simulink model "NED_INS_V2"  (R2020a)
settings: Solver=FixedStepDiscrete  StartTime=0.0  StopTime=60  FixedStep=0.01  RelTol=1e-3
InitFcn:
  | INS_sample_time=0.01;
  | load('GPS1hz_INS_Car_60s.mat')
settings Model: Creator=Toranj  LastModifiedBy=Toranj

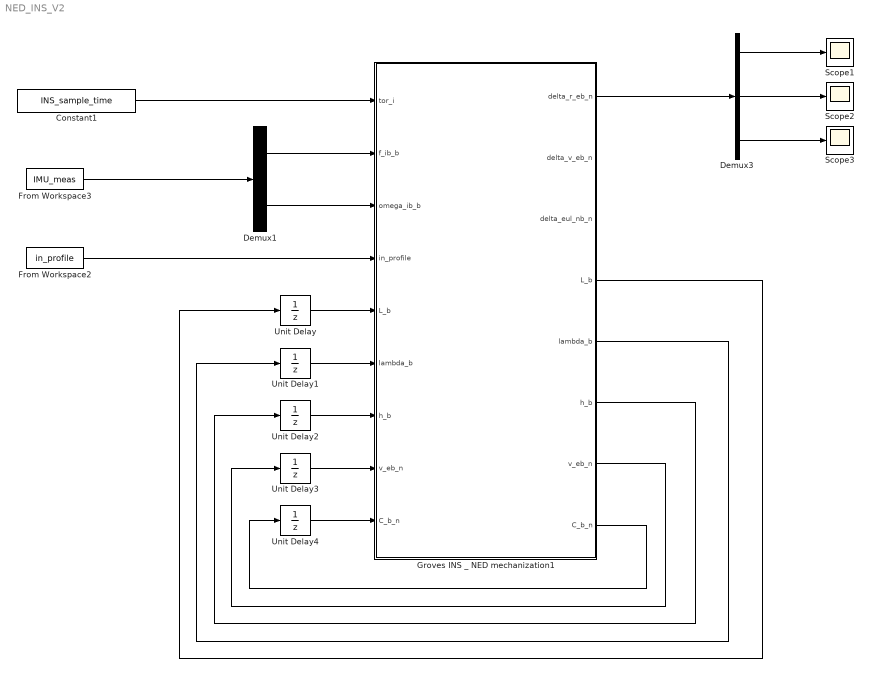
== system NED_INS_V2 ==
  Constant1 : Constant  Value=INS_sample_time
  Demux1 : Demux  Outputs=2
  Demux3 : Demux  Outputs=3
  From Workspace2 : FromWorkspace  VariableName=in_profile
  From Workspace3 : FromWorkspace  VariableName=IMU_meas
  Groves INS _ NED mechanization1 : MATLAB Function  TreatAsAtomicUnit=on  mask{old_true_L_b=0.890117918520000, old_true_lambda_b=0, old_true_h_b=10, old_true_v_eb_n=[0;0;0], old_true_C_b_n=eye(3)}
      mask prompts: old_true_L_b "Init_L_b"; old_true_lambda_b "Init_lambda_b"; old_true_h_b "Init_h_b"; old_true_v_eb_n "Init_v_eb_n"; old_true_C_b_n "Init_true_C_b_n"
      mask init:
      | deg_to_rad = 0.01745329252;
      | % rad_to_deg = 1/deg_to_rad;
      | % micro_g_to_meters_per_second_squared = 9.80665E-6;
      | 
      | % Position initialization error (m; N,E,D)
      | initialization_errors.delta_r_eb_n = [4;2;3];
      | % Velocity initialization error (m/s; N,E,D)
      | initialization_errors.delta_v_eb_n = [0.05;-0.05;0.1];
      | % Attitude initialization error (deg, converted to rad; @N,E,D)
      | initialization_errors.delta_eul_nb_n = [-0.05;0.04;1]*deg_to_rad; % rad
      | 
      | [L_b0,lambda_b0,h_b0,v_eb_n0,C_b_n0] =...
      |     Initialize_NED(old_true_L_b,old_true_lambda_b,old_true_h_b,...
      |     old_true_v_eb_n,old_true_C_b_n,initialization_errors);
  Scope1 : Scope
  Scope2 : Scope
  Scope3 : Scope
  Unit Delay : UnitDelay  InitialCondition=0.890117918520000  SampleTime=-1  HasFrameUpgradeWarning=on
  Unit Delay1 : UnitDelay  SampleTime=-1  HasFrameUpgradeWarning=on
  Unit Delay2 : UnitDelay  InitialCondition=10  SampleTime=-1  HasFrameUpgradeWarning=on
  Unit Delay3 : UnitDelay  InitialCondition=[0;0;0]  SampleTime=-1  HasFrameUpgradeWarning=on
  Unit Delay4 : UnitDelay  InitialCondition=eye(3)  SampleTime=-1  HasFrameUpgradeWarning=on
  wires:
  From Workspace2/1 -> Groves INS _ NED mechanization1/4(in_profile)
  Constant1/1 -> Groves INS _ NED mechanization1/1(tor_i)
  Demux1/1 -> Groves INS _ NED mechanization1/2(f_ib_b)
  From Workspace3/1 -> Demux1/1
  Unit Delay/1 -> Groves INS _ NED mechanization1/5("L_b ")
  Groves INS _ NED mechanization1/5(lambda_b) -> Unit Delay1/1
  Unit Delay2/1 -> Groves INS _ NED mechanization1/7("h_b ")
  Groves INS _ NED mechanization1/4(L_b) -> Unit Delay/1
  Groves INS _ NED mechanization1/8(C_b_n) -> Unit Delay4/1
  Unit Delay3/1 -> Groves INS _ NED mechanization1/8("v_eb_n ")
  Groves INS _ NED mechanization1/6(h_b) -> Unit Delay2/1
  Unit Delay1/1 -> Groves INS _ NED mechanization1/6("lambda_b ")
  Groves INS _ NED mechanization1/7(v_eb_n) -> Unit Delay3/1
  Unit Delay4/1 -> Groves INS _ NED mechanization1/9("C_b_n ")
  Demux1/2 -> Groves INS _ NED mechanization1/3(omega_ib_b)
  Demux3/3 -> Scope3/1
  Demux3/2 -> Scope2/1
  Demux3/1 -> Scope1/1
  Groves INS _ NED mechanization1/1(delta_r_eb_n) -> Demux3/1

== matlab function NED_INS_V2/Groves INS _ NED mechanization1 ==
  data: delta_r_eb_n output; delta_v_eb_n output; delta_eul_nb_n output; tor_i input; L_b output; f_ib_b input; omega_ib_b input; in_profile input; lambda_b output; h_b output; v_eb_n output; C_b_n output; L_b input; lambda_b input; h_b input; v_eb_n input; C_b_n input
% function [L_b,lambda_b,h_b,v_eb_n,C_b_n] = Nav_equations_NED(tor_i,...
%         old_L_b,old_lambda_b,old_h_b,old_v_eb_n,old_C_b_n,f_ib_b,omega_ib_b)
function [delta_r_eb_n,delta_v_eb_n,delta_eul_nb_n,L_b,lambda_b,h_b,v_eb_n,C_b_n] = Nav_equations_NED(tor_i,...
    f_ib_b,omega_ib_b,in_profile,L_b,lambda_b,h_b,v_eb_n,C_b_n)
%Nav_equations_NED - Runs precision local-navigation-frame inertial
%navigation equations (Note: only the attitude update and specific force
%frame transformation phases are precise.)
%
% Software for use with "Principles of GNSS, Inertial, and Multisensor
% Integrated Navigation Systems," Second Edition.
%
% This function created 1/4/2012 by Paul Groves
%
% Inputs:
%   tor_i         time interval between epochs (s)
%   old_L_b       previous latitude (rad)
%   old_lambda_b  previous longitude (rad)
%   old_h_b       previous height (m)
%   old_C_b_n     previous body-to-NED coordinate transformation matrix
%   old_v_eb_n    previous velocity of body frame w.r.t. ECEF frame, resolved
%                 along north, east, and down (m/s)
%   f_ib_b        specific force of body frame w.r.t. ECEF frame, resolved
%                 along body-frame axes, averaged over time interval (m/s^2)
%   omega_ib_b    angular rate of body frame w.r.t. ECEF frame, resolved
%                 about body-frame axes, averaged over time interval (rad/s)
% Outputs:
%   L_b           latitude (rad)
%   lambda_b      longitude (rad)
%   h_b           height (m)
%   v_eb_n        velocity of body frame w.r.t. ECEF frame, resolved along
%                 north, east, and down (m/s)
%   C_b_n         body-to-NED coordinate transformation matrix

% Copyright 2012, Paul Groves
% License: BSD; see license.txt for details

% parameters
omega_ie = 7.292115E-5;  % Earth rotation rate (rad/s)

% Begins
% persistent old_L_b old_lambda_b old_h_b old_v_eb_n old_C_b_n;
% if isempty(old_L_b)
%     old_L_b = L_b0;
%     old_lambda_b = lambda_b0;
%     old_h_b = h_b0;
%     old_v_eb_n = v_eb_n0;
%     old_C_b_n = C_b_n0;
% end
% PRELIMINARIES
% Calculate attitude increment, magnitude, and skew-symmetric matrix

    old_L_b = L_b;
    old_lambda_b = lambda_b;
    old_h_b = h_b;
    old_v_eb_n = v_eb_n;
    old_C_b_n = C_b_n;

alpha_ib_b = omega_ib_b * tor_i;
mag_alpha = sqrt(alpha_ib_b' * alpha_ib_b);
Alpha_ib_b = Skew_symmetric(alpha_ib_b);

% From (2.123) , determine the angular rate of the ECEF frame
% w.r.t the ECI frame, resolved about NED
omega_ie_n = omega_ie * [cos(old_L_b); 0; - sin(old_L_b)];

% From (5.44), determine the angular rate of the NED frame
% w.r.t the ECEF frame, resolved about NED
[old_R_N,old_R_E] = Radii_of_curvature(old_L_b);
old_omega_en_n = [old_v_eb_n(2) / (old_R_E + old_h_b);...
    -old_v_eb_n(1) / (old_R_N + old_h_b);...
    -old_v_eb_n(2) * tan(old_L_b) / (old_R_E + old_h_b)];

% SPECIFIC FORCE FRAME TRANSFORMATION
% Calculate the average body-to-ECEF-frame coordinate transformation
% matrix over the update interval using (5.84) and (5.86)
if mag_alpha>1.E-8
    ave_C_b_n = old_C_b_n * (eye(3) + (1 - cos(mag_alpha)) / mag_alpha^2 ...
        * Alpha_ib_b + (1 - sin(mag_alpha) / mag_alpha) / mag_alpha^2 ...
        * Alpha_ib_b * Alpha_ib_b) -...
        0.5 * Skew_symmetric(old_omega_en_n + omega_ie_n) * old_C_b_n;
else
    ave_C_b_n = old_C_b_n -...
        0.5 * Skew_symmetric(old_omega_en_n + omega_ie_n) * old_C_b_n;
end %if mag_alpha

% Transform specific force to ECEF-frame resolving axes using (5.86)
f_ib_n = ave_C_b_n * f_ib_b;

% UPDATE VELOCITY
% From (5.54),
v_eb_n = old_v_eb_n + tor_i * (f_ib_n + Gravity_NED(old_L_b,old_h_b) -...
    Skew_symmetric(old_omega_en_n + 2 * omega_ie_n) * old_v_eb_n);

% UPDATE CURVILINEAR POSITION
% Update height using (5.56)
h_b = old_h_b - 0.5 * tor_i * (old_v_eb_n(3) + v_eb_n(3));

% Update latitude using (5.56)
L_b = old_L_b + 0.5 * tor_i * (old_v_eb_n(1) / (old_R_N + old_h_b) +...
    v_eb_n(1) / (old_R_N + h_b));

% Calculate meridian and transverse radii of curvature
[R_N,R_E]= Radii_of_curvature(L_b);

% Update longitude using (5.56)
lambda_b = old_lambda_b + 0.5 * tor_i * (old_v_eb_n(2) / ((old_R_E +...
    old_h_b) * cos(old_L_b)) + v_eb_n(2) / ((R_E + h_b) * cos(L_b)));

% ATTITUDE UPDATE
% From (5.44), determine the angular rate of the NED frame
% w.r.t the ECEF frame, resolved about NED
omega_en_n = [v_eb_n(2) / (R_E + h_b);...
    -v_eb_n(1) / (R_N + h_b);...
    -v_eb_n(2) * tan(L_b) / (R_E + h_b)];

% Obtain coordinate transformation matrix from the new attitude w.r.t. an
% inertial frame to the old using Rodrigues' formula, (5.73)
if mag_alpha>1.E-8
    C_new_old = eye(3) + sin(mag_alpha) / mag_alpha * Alpha_ib_b +...
        (1 - cos(mag_alpha)) / mag_alpha^2 * Alpha_ib_b * Alpha_ib_b;
else
    C_new_old = eye(3) + Alpha_ib_b;
end %if mag_alpha

% Update attitude using (5.77)
C_b_n = (eye(3) - Skew_symmetric(omega_ie_n + 0.5 * omega_en_n + 0.5 *...
    old_omega_en_n)  * tor_i) * old_C_b_n * C_new_old;



true_L_b = in_profile(1);
true_lambda_b = in_profile(2);
true_h_b = in_profile(3);
true_v_eb_n = in_profile(4:6);
true_eul_nb = in_profile(7:9);
true_C_b_n = Euler_to_CTM(true_eul_nb)';
[delta_r_eb_n,delta_v_eb_n,delta_eul_nb_n] = Calculate_errors_NED(...
    L_b,lambda_b,h_b,v_eb_n,C_b_n,true_L_b,...
    true_lambda_b,true_h_b,true_v_eb_n,true_C_b_n);

old_L_b = L_b;
old_lambda_b = lambda_b;
old_h_b = h_b;
old_v_eb_n = v_eb_n;
old_C_b_n = C_b_n;
% Ends
